simulink model "Practica_1"  (R2022b)
settings: Solver=VariableStepAuto  StartTime=0.0  StopTime=10.0  MaxStep=0.00001  RelTol=1e-3
values from neighbouring files (symbols this model uses):
  g = 9.81    [Parametros_Practica1.m]    (also in Practica2.m)
  l1 = 0.3    [Parametros_Practica1.m]    (also in Practica2.m)
  l2 = 0.25    [Parametros_Practica1.m]    (also in Practica2.m)
  m1 = 290    [CuartoSuspension.m]    (also in Parametros_Practica1.m = 0.2; Practica2.m = 0.1; variablespractica3.m)
  m2 = 59    [CuartoSuspension.m]    (also in Parametros_Practica1.m = 0.1; Practica2.m = 0.1; variablespractica3.m)
settings Model: Creator=52466  LastModifiedBy=52466

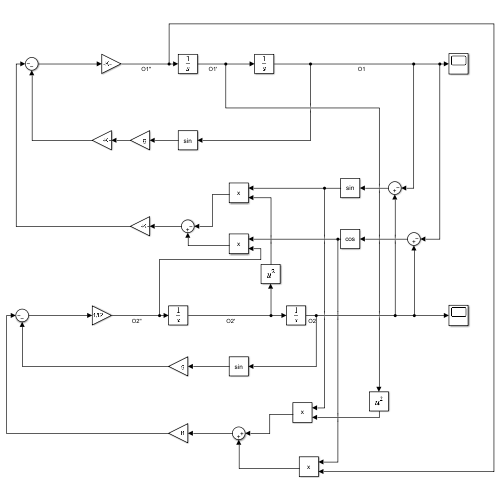
[thumbnail: Simulink's stored preview of the top-level diagram]
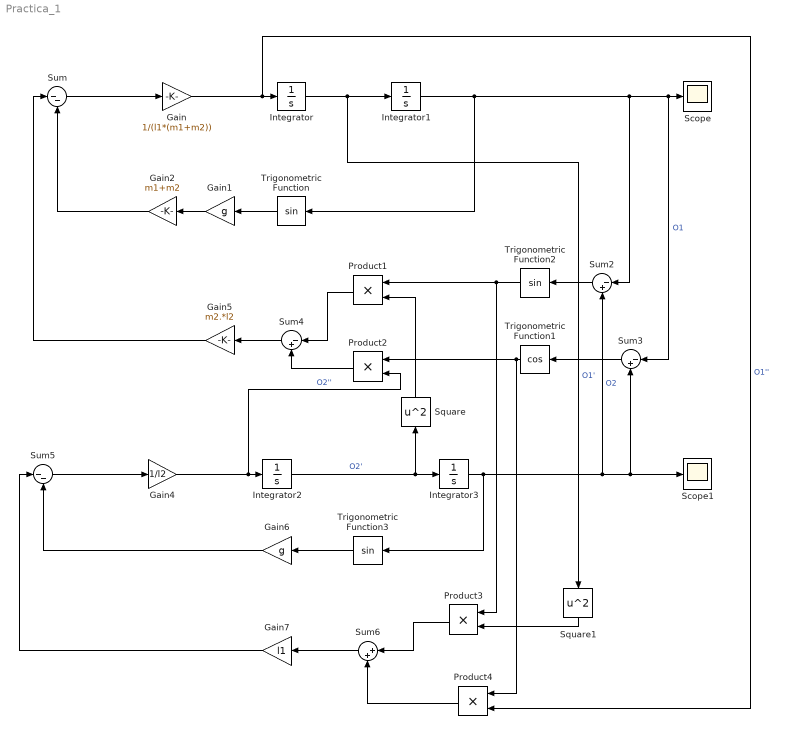
== system Practica_1 ==
  Gain : Gain  Gain=1/(l1*(m1+m2))
  Gain1 : Gain  Gain=g
  Gain2 : Gain  Gain=m1+m2
  Gain4 : Gain  Gain=1/l2
  Gain5 : Gain  Gain=m2.*l2
  Gain6 : Gain  Gain=g
  Gain7 : Gain  Gain=l1
  Integrator : Integrator
  Integrator1 : Integrator
  Integrator2 : Integrator
  Integrator3 : Integrator  InitialCondition=35*(pi/180)
  Product{1..4} (4 alike) : Product
  Scope : Scope
  Scope1 : Scope
  Square : Math  Operator=square
  Square1 : Math  Operator=square
  Sum : Sum  Inputs=|--
  Sum2 : Sum  Inputs=|-+
  Sum3 : Sum  Inputs=|-+
  Sum4 : Sum  Inputs=|-+
  Sum5 : Sum  Inputs=|--
  Sum6 : Sum  Inputs=|++
  Trigonometric Function : Trigonometry
  Trigonometric Function1 : Trigonometry  Operator=cos
  Trigonometric Function2 : Trigonometry
  Trigonometric Function3 : Trigonometry
  wires:
  Integrator/1 -> Square1/1, Integrator1/1  "O1'"
  Gain/1 -> Product4/2, Integrator/1  "O1''"
  Trigonometric Function/1 -> Gain1/1
  Sum/1 -> Gain/1
  Integrator1/1 -> Trigonometric Function/1, Sum2/1, Sum3/1, Scope/1  "O1"
  Gain2/1 -> Sum/2
  Sum2/1 -> Trigonometric Function2/1
  Sum3/1 -> Trigonometric Function1/1
  Gain6/1 -> Sum5/2
  Sum5/1 -> Gain4/1
  Integrator3/1 -> Sum3/2, Scope1/1, Sum2/2, Trigonometric Function3/1  "O2"
  Gain4/1 -> Product2/2, Integrator2/1  "O2''"
  Integrator2/1 -> Square/1, Integrator3/1  "O2'"
  Square/1 -> Product1/2
  Product1/1 -> Sum4/1
  Product2/1 -> Sum4/2
  Trigonometric Function1/1 -> Product4/1, Product2/1
  Sum4/1 -> Gain5/1
  Gain5/1 -> Sum/1
  Trigonometric Function3/1 -> Gain6/1
  Product4/1 -> Sum6/2
  Product3/1 -> Sum6/1
  Square1/1 -> Product3/2
  Trigonometric Function2/1 -> Product3/1, Product1/1
  Sum6/1 -> Gain7/1
  Gain7/1 -> Sum5/1
  Gain1/1 -> Gain2/1
